simulink model "system_3dof"  (R2025b)
settings: Solver=FixedStepAuto  StartTime=0.0  StopTime=60  FixedStep=0.005  RelTol=1e-3
InitFcn:
  | params_3dof
settings Model: Creator=schwmaxi  LastModifiedBy=schwmaxi
settings DataIOCC: SaveFormat=Structure  SaveTime=off
settings OptimizationCC: UseDivisionForNetSlopeComputation=on  GainParamInheritBuiltInType=on  UseFloatMulNetSlope=on  EnhancedBackFolding=on  BooleansAsBitfields=on  PassReuseOutputArgsAs=Individual arguments  StateBitsets=on  DataBitsets=on  ZeroExternalMemoryAtStartup=off  ZeroInternalMemoryAtStartup=off  NoFixptDivByZeroProtection=on  EfficientFloat2IntCast=on  LifeSpan=1  OptimizeBlockOrder=speed  DifferentSizesBufferReuse=on  EfficientTunableParamExpr=on
settings DebuggingCC: ParameterTunabilityLossMsg=error
settings HardwareCC: ProdBitPerPointer=32.0  ProdBitPerSizeT=32.0  ProdBitPerPtrDiffT=32.0  ProdLargestAtomicFloat=None  ProdWordSize=32.0  ProdLongLongMode=on  ProdHWDeviceType=Custom Processor->Custom Processor
settings SFSimCC: MATLABDynamicMemAlloc=off  SimTargetLang=C++  SimDLTargetLibrary=mkl-dnn
settings RTWCC: SystemTargetFile=ert.tlc  GenCodeOnly=on  TemplateMakefile=ert_default_tmf  TargetLang=C++  Description=Embedded Coder
settings CodeAppCC: ForceParamTrailComments=on  IgnoreCustomStorageClasses=off  OperatorAnnotations=on  SimulinkDataObjDesc=on  SFDataObjDesc=on  CustomSymbolStrGlobalVar=rt$N$M  CustomSymbolStrType=$N$M  CustomSymbolStrFcn=$N$M$F  CustomSymbolStrMacro=$N$M  InsertBlockDesc=on
settings ERTTargetCC: InlinedParameterPlacement=Hierarchical  RootIOFormat=Structure reference  ERTCustomFileTemplate=example_file_process.tlc  ERTFilePackagingFormat=CompactWithDataFile  TargetLangStandard=C++11 (ISO)  GenerateSampleERTMain=on  IncludeMdlTerminateFcn=off  CombineSignalStateStructs=on  SupportAbsoluteTime=off  CodeInterfacePackaging=C++ class  SubcomponentCodeInterfacePackaging=C++ class  SupportComplex=off  SupportNonInlinedSFcns=on

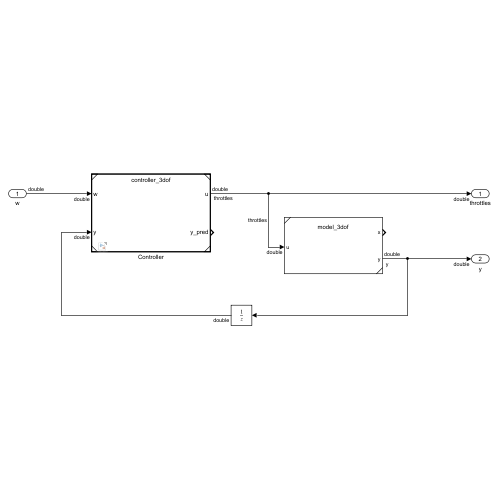
[thumbnail: Simulink's stored preview of the top-level diagram]
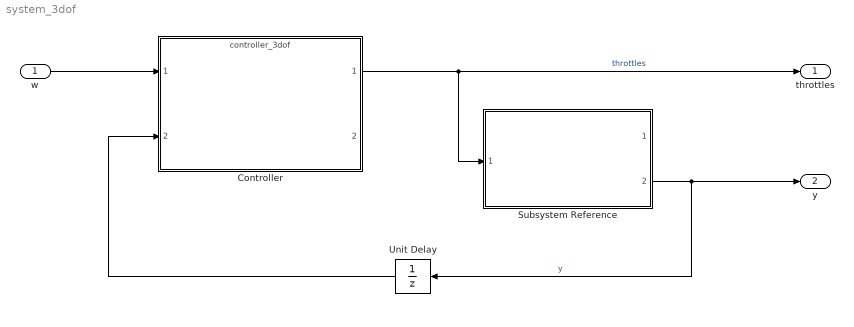
== system system_3dof ==
  w : Inport  OutDataTypeStr=double  PortDimensions=4
  Controller : ModelReference  ModelNameDialog=controller_3dof.slx  SimulationMode=Normal  ModelReferenceVersion=1.273
  Subsystem Reference : Subsystem  ReferencedSubsystem=model_3dof
  Unit Delay : UnitDelay  SampleTime=-1  HasFrameUpgradeWarning=on
  throttles : Outport  OutDataTypeStr=double  PortDimensions=[4 1]  SampleTime=0
  y : Outport  Port=2  OutDataTypeStr=double  PortDimensions=3  SampleTime=0
  wires:
  Controller/1 -> Subsystem Reference/1, throttles/1  "throttles"
  Subsystem Reference/2 -> Unit Delay/1, y/1  "y"
  Unit Delay/1 -> Controller/2
  w/1 -> Controller/1
